simulink model "rehastim_gui"  (R2014b)
settings: Solver=FixedStepDiscrete  StartTime=0.0  StopTime=inf  FixedStep=0.01  RelTol=1e-3
undefined symbols (not defined in the file or in its folder): rehastim_config
libraries: PaPI x1
settings Model: SimulationMode=external  Creator=sven  LastModifiedBy=sven
settings OptimizationCC: OptimizeModelRefInitCode=on  LifeSpan=Inf
settings DebuggingCC: UnderspecifiedInitializationDetection=Classic  MergeDetectMultiDrivingBlocksExec=none  InheritedTsInSrcMsg=none  StateNameClashWarn=warning
settings RTWCC: SystemTargetFile=ert_linux.tlc  MakeCommand="make_rtw OPT_OPTS=\"-DWITH_HW\""  TemplateMakefile=ert_linux.tmf  Description=Linux Embedded Coder  ProcessScript=ert_linux_make_rtw_hook  TargetLang=C++
settings RTWCC: CustomInclude=|
  | /usr/local/MATLAB/R2014b/sys/os/glnxa64/
  | /usr/lib/x86_64-linux-gnu/
  | /usr/include/
settings RTWCC: CustomLibrary=|
  | libstdc++.so.6
  | libgcc_s.so.1
  | libgfortran.so.3
  | libdl.so
  | libboost_system.so
  | libboost_thread.so
  | libboost_signals.so
settings CodeAppCC: IgnoreCustomStorageClasses=off
settings STFCustomTargetCC: ModelReferenceCompliant=off  CombineOutputUpdateFcns=on  ERTCustomFileBanners=on  SupportContinuousTime=off  SupportNonInlinedSFcns=off  MATLABClassNameForMDSCustomization=Simulink.SoftwareTarget.ERTCustomization  GRTInterface=off  SystemTargetFile=ert_linux.tlc
settings ERTTargetCC: ModelReferenceCompliant=off  ParMdlRefBuildCompliant=off  CompOptLevelCompliant=off  ConcurrentExecutionCompliant=off  ERTFirstTimeCompliant=off  ModelStepFunctionPrototypeControlCompliant=off  CPPClassGenCompliant=off  ExtMode=on  InlinedParameterPlacement=NonHierarchical  ERTCustomFileTemplate=ert_linux_file_process.tlc

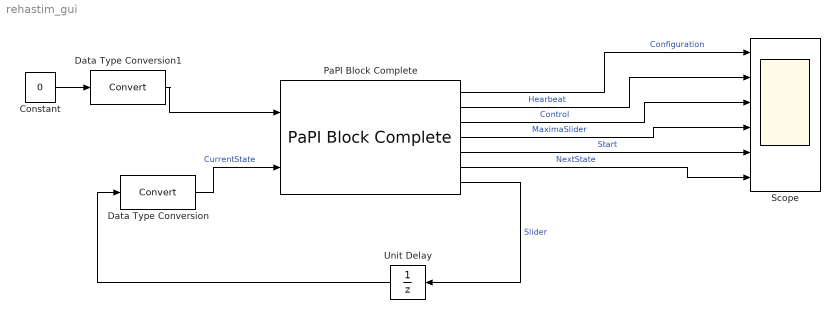
== system rehastim_gui ==
  Constant : Constant  Value=0
  Data Type Conversion : DataTypeConversion
  Data Type Conversion1 : DataTypeConversion
  PaPI Block Complete : PaPI/PaPI Block Complete  amount_parameters=[45,1,1,8,1,1,1]  define_inputs=[1]  split_inputs=[1]  json_string=rehastim_config(1)  UDPLocalPort=20001  UDPRemotePort=20000  UDPRemoteIP='127.0.0.1'  output_size=700  UDPStart=on  sample_time=-1
  Scope : Scope  NumInputPorts=6
      settings: TimeRange=10  YMin=0~1~-1~-1~-1~1  YMax=80~2~1~1~1~3  MaxDataPoints=50000
  Unit Delay : UnitDelay  SampleTime=-1
  wires:
  PaPI Block Complete/1 -> Scope/1  "Configuration"
  PaPI Block Complete/2 -> Scope/2  "Hearbeat"
  PaPI Block Complete/3 -> Scope/3  "Control"
  PaPI Block Complete/4 -> Scope/4  "MaximaSlider"
  Unit Delay/1 -> Data Type Conversion/1
  Data Type Conversion/1 -> PaPI Block Complete/2  "CurrentState"
  Constant/1 -> Data Type Conversion1/1
  Data Type Conversion1/1 -> PaPI Block Complete/1
  PaPI Block Complete/5 -> Scope/5  "Start"
  PaPI Block Complete/6 -> Scope/6  "NextState"
  PaPI Block Complete/7 -> Unit Delay/1  "Slider"
